simulink library "DMS_slave_lib"  (Simulink 8.1)
settings: Solver=ode45  StartTime=0.0  StopTime=10.0  RelTol=1e-3
libraries: rtio_generic_modbus x1
settings Model: Creator=ch24070  LastModifiedBy=ch24070

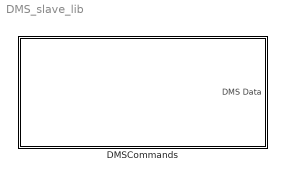
== system DMS_slave_lib ==
  DMSCommands : Subsystem

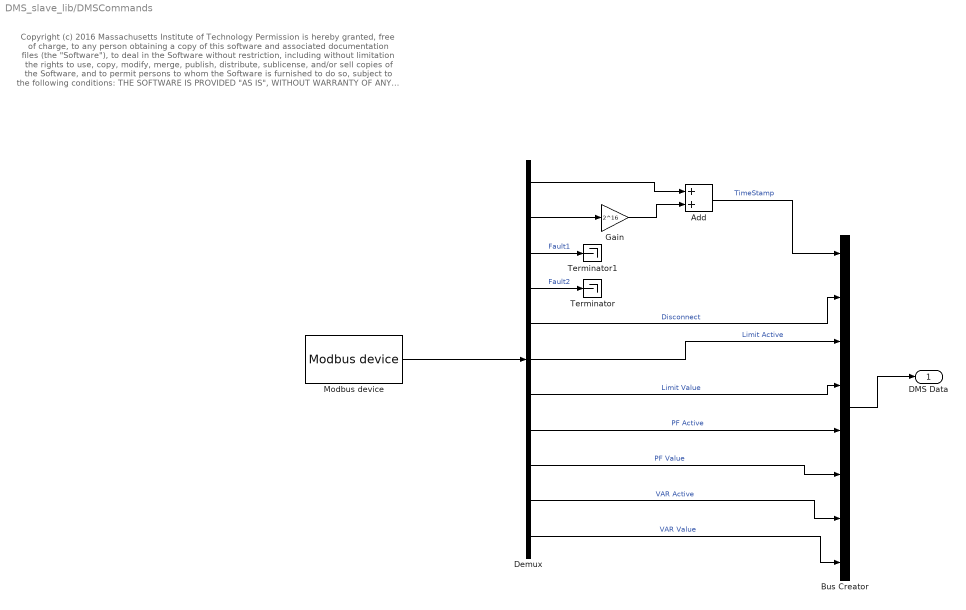
== system DMS_slave_lib/DMSCommands ==
  note: Copyright (c) 2016 Massachusetts Institute of Technology
      | Permission is hereby granted, free of charge, to any person obtaining a copy of this software and associated documentation files (the "Software"), to deal
      | in the Software without restriction, including without limitation the rights to use, copy, modify, merge, publish, distribute, sublicense, and/or sell copies of the
      | Software, and to permit persons to whom the Software is furnished to do so, subject to the following conditions:
      |
      | THE SOFTWARE IS PROVIDED "AS IS", WITHOUT WARRANTY OF ANY KIND, EXPRESS OR IMPLIED, INCLUDING BUT NOT LIMITED TO THE
      | WARRANTIES OF MERCHANTABILITY, FITNESS FOR A PARTICULAR PURPOSE AND NONINFRINGEMENT. IN NO EVENT SHALL THE AUTHORS
      | OR COPYRIGHT HOLDERS BE LIABLE FOR ANY CLAIM, DAMAGES OR OTHER LIABILITY, WHETHER IN AN ACTION OF CONTRACT, TORT OR
      | OTHERWISE, ARISING FROM, OUT OF OR IN CONNECTION WITH THE SOFTWARE OR THE USE OR OTHER DEALINGS IN THE SOFTWARE
  Add : Sum
  Bus Creator : BusCreator  Inputs=8
  Demux : Demux  Outputs=11
  Gain : Gain  Gain=2^16
  Modbus device : rtio_generic_modbus/Modbus device  conf_name=DMS_cfg.opal  conf_name_mask=DMS_cfg.xls  sample_time=Ts
  Terminator : Terminator
  Terminator1 : Terminator
  DMS Data : Outport
  wires:
  Add/1 -> Bus Creator/1  "TimeStamp"
  Demux/1 -> Add/1
  Demux/2 -> Gain/1
  Gain/1 -> Add/2
  Modbus device/1 -> Demux/1
  Bus Creator/1 -> DMS Data/1
  Demux/5 -> Bus Creator/2  "Disconnect"
  Demux/6 -> Bus Creator/3  "Limit Active"
  Demux/7 -> Bus Creator/4  "Limit Value"
  Demux/4 -> Terminator/1  "Fault2"
  Demux/3 -> Terminator1/1  "Fault1"
  Demux/8 -> Bus Creator/5  "PF Active"
  Demux/9 -> Bus Creator/6  "PF Value"
  Demux/10 -> Bus Creator/7  "VAR Active"
  Demux/11 -> Bus Creator/8  "VAR Value"
